simulink model "model_socrates"  (R2019b)
settings: Solver=VariableStepAuto  StartTime=0.0  StopTime=nb_time_unit_in_a_simulation/5  RelTol=1e-3
values from neighbouring files (symbols this model uses):
  nb_air_cons = nb_rooms-2    [load_parameters.m]
  nb_boilers = 2    [load_parameters.m]
  nb_radiators = nb_rooms-2    [load_parameters.m]
  nb_second_in_timeunit = 60*5    (= 300)    [full_test.m]
  nb_step_to_fifteen_min = 3    [full_test.m]
  nb_step_to_one_h = 12    [full_test.m]
  nb_step_to_thirty_min = 6    [full_test.m]
  timeunit_in_a_day = 2*6*24    (= 288)    [full_test.m]
undefined symbols (not defined in the file or in its folder): air_mass_kg_rooms, Area_boiler, area_outdoor_rooms, Area_radiators, area_rooms_ground, area_walls_between_rooms, C_air, C_water, Energy_used_by_air_conditioner_for_1_timeunit_in_Watts_vector, Energy_used_by_air_mixer_for_1_timeunit_in_Watts, Energy_used_by_boiler_for_1_timeunit_in_Watts, initial_relative_humidity, initial_temp_water_in_boilers, initial_temperature_rooms, initial_temperature_water_in_radiator, k_boiler_border, k_radiators, k_wall_outdoor_rooms, k_walls_between_rooms, mass_water_radiator, matrix_AC_rooms_locations, matrix_boiler_radiator_connection, matrix_boiler_rooms_locations, matrix_radiator_rooms_locations, nb_humans, nb_rooms, outdoor_max_temp_A, outdoor_max_temp_B, outdoor_min_temp_A, outdoor_min_temp_B, tau_boiler, thickness_boiler, thickness_outdoor_rooms, thickness_radiator_pipes, thickness_walls_between_rooms, Volume_radiators, Volume_rooms, water_weight_in_boiler, watt_generation_of_employe
libraries: dspmtrx3 x15, dspstat3 x6, simulink x2
(part 1 of 2)
settings Model: Creator=pat  LastModifiedBy=pat

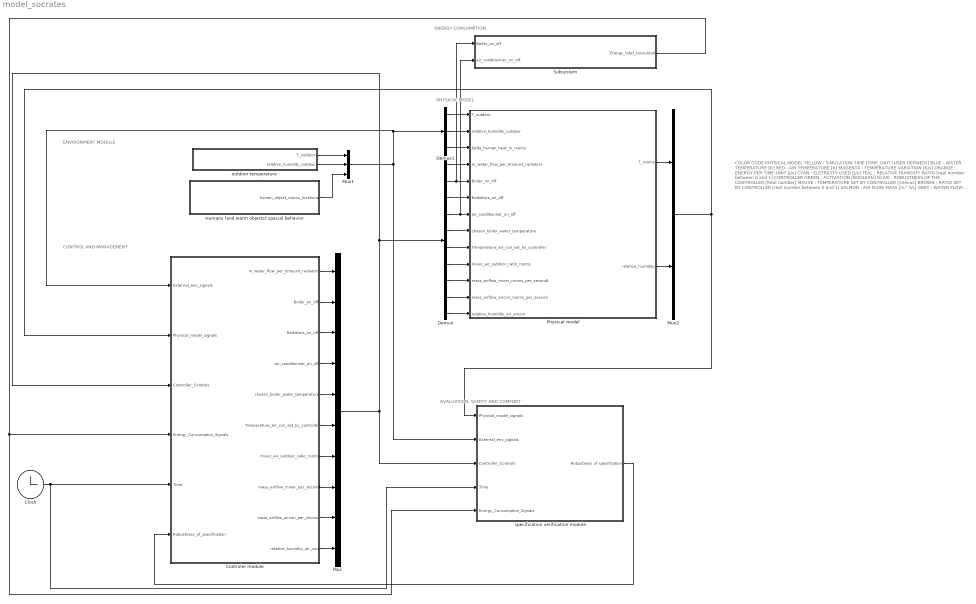
== system model_socrates ==
  note: EVALUATION, SAFETY AND COMFORT
  note: PHYSICAL MODEL
  note: ENVIRONMENT MODULE
  note: COLOR CODE
      |
      | PHYSICAL MODEL
      |
      | YELLOW : SIMULATION TIME [TIME_UNIT (USER DEFINED)]
      | BLUE : WATER TEMPERATURE [K]
      | RED : AIR TEMPERATURE [K]
      | MAGENTA : TEMPERATURE VARIATION [K/s]
      | ORANGE : ENERGY PER TIME-UNIT [J/s]
      | CYAN : ELETRICITY USED [J/s]
      | TEAL : RELATIVE HUMIDITY RATIO [real number between 0 and 1]
      |
      | CONTROLLER
      |
      | GREEN : ACTIVATION [BOOLEAN]
      | OLIVE : ROBUSTNESS OF THE CONTROLLER [Real number]
      | MAUVE : TEMPERATURE SET BY CONTROLLER [Celsius]
      | BROWN : RATIO SET BY CONTROLLER [real number between 0 and 1]
      | SALMON : AIR FLOW MASS [m^3/s]
      | GREY : WATER FLOW MASS [m^3/s]
      |
      | ENVIRONMENT STOCHASTIC BEHAVIORS
      |
      | PURPLE : WARM HUMAN AND OBJECTS LOCATION
      | : POSSESES SOME STOCHASTIC BEHAVIORS
  note: CONTROL AND MANAGEMENT
  note: ENERGY CONSUMPTION
  Clock : Clock
  Controler module : Subsystem
  Demux : Demux  Outputs=[nb_radiators nb_boilers nb_radiators nb_air_cons nb_boilers nb_air_cons nb_rooms nb_rooms nb_air_cons nb_air_cons]
  Demux1 : Demux  Outputs=[1 1 nb_humans]
  "Humans (and warm objects) spacial behavior " : Subsystem
  Mux : Mux  Inputs=10
  Mux1 : Mux  Inputs=3
  Mux2 : Mux  Inputs=2
  Physical model : Subsystem
  Subsystem : Subsystem
  outdoor temperature : Subsystem
  specification verification module : Subsystem
  wires:
  specification verification module/1(Robustness of spesification) -> Controler module/6(Robustness_of_specification)
  Physical model/2(relative_humidity) -> Mux2/2
  Controler module/1(m_water_flow_per_timeunit_radiators) -> Mux/1
  Controler module/2(Boiler_on_off) -> Mux/2
  Controler module/3(Radiators_on_off) -> Mux/3
  Controler module/4(air_conditionner_on_off) -> Mux/4
  Controler module/5(chosen_boiler_water_temperature) -> Mux/5
  Controler module/6(Temperature_air_con_set_by_controller) -> Mux/6
  Controler module/7("mixer_air_outdoor_ratio_rooms ") -> Mux/7
  Controler module/8(mass_airflow_mixer_per_second) -> Mux/8
  Controler module/9(mass_airflow_aircon_per_second) -> Mux/9
  Controler module/10(relative_humidity_air_con) -> Mux/10
  Demux/1 -> Physical model/4(m_water_flow_per_timeunit_radiators)
  Demux/3 -> Physical model/6(Radiators_on_off)
  Demux/10 -> Physical model/13(relative_humidity_air_aircon)
  Demux/9 -> Physical model/12(mass_airflow_aircon_rooms_per_second)
  Demux/8 -> Physical model/11(mass_airflow_mixer_rooms_per_secondt)
  Demux/7 -> Physical model/10("mixer_air_outdoor_ratio_rooms ")
  Demux/6 -> Physical model/9(Temperature_air_con_set_by_controller)
  Demux/5 -> Physical model/8(chosen_boiler_water_temperature)
  Clock/1 -> Controler module/5(Time), specification verification module/4(Time)
  "Humans (and warm objects) spacial behavior "/1("human_object_rooms_locations ") -> Mux1/3
  outdoor temperature/2("relative_humidity_outdoor ") -> Mux1/2
  outdoor temperature/1(T_outdoor) -> Mux1/1
  Demux1/1 -> Physical model/1(T_outdoor)
  Demux1/3 -> Physical model/3("Delta_human_heat_in_rooms ")
  Demux1/2 -> Physical model/2(relative_humidity_outdoor)
  Subsystem/1(Energy_total_consumed) -> specification verification module/5(Energy_Consumption_Signals), Controler module/4(Energy_Consumption_Signals)
  Physical model/1(T_rooms) -> Mux2/1
  Mux2/1 -> Controler module/2(Physical_model_signals), specification verification module/1(Physical_model_signals)
  Mux1/1 -> Controler module/1(External_env_signals), Demux1/1, specification verification module/2(External_env_signals)
  Mux/1 -> Controler module/3("Controller_Controls "), Demux/1, specification verification module/3("Controller_Controls ")
  Demux/2 -> Subsystem/1(Boiler_on_off), Physical model/5(Boiler_on_off)
  Demux/4 -> Subsystem/2(air_conditionner_on_off), Physical model/7(air_conditionner_on_off)

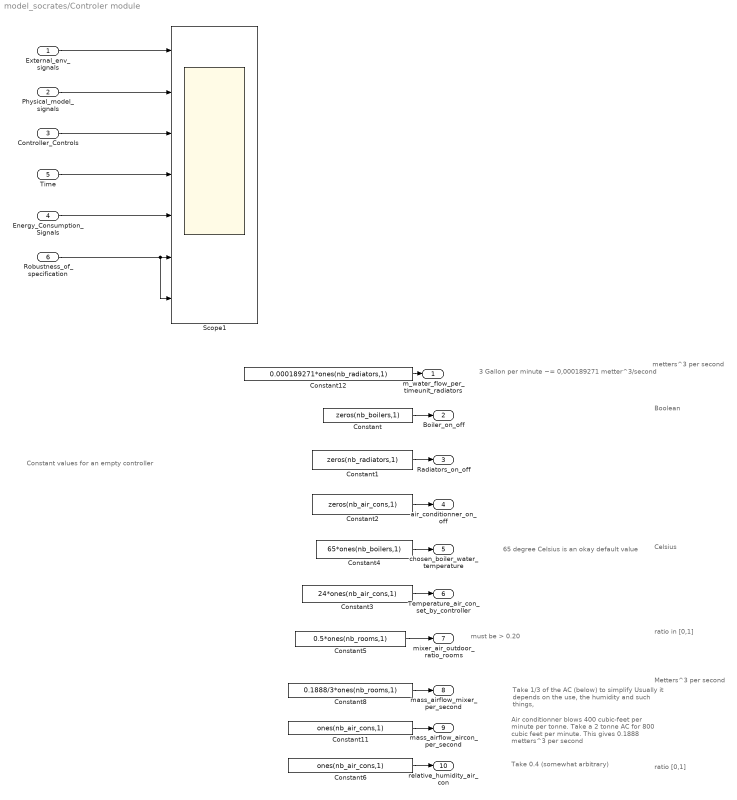
== system model_socrates/Controler module ==
  note: Metters^3 per second
  note: Air conditionner blows 400 cubic-feet per minute per tonne. Take a 2 tonne AC for 800 cubic feet per minute.
      |
      | This gives 0.1888 metters^3 per second
  note: 3 Gallon per minute ~= 0,000189271 metter^3/second
  note: 65 degree Celsius is an okay default value
  note: Constant values
      | for an empty controller
  note: must be > 0.20
  note: Take 1/3 of the AC (below) to simplify
      | Usually it depends on the use, the humidity
      | and such things,
  note: ratio in [0,1]
  note: Celsius
  note: Boolean
  note: metters^3 per second
  note: Take 0.4 (somewhat arbitrary)
  note: ratio [0,1]
  External_env_signals : Inport
  Physical_model_signals : Inport  Port=2
  "Controller_Controls " : Inport  Port=3
  Energy_Consumption_Signals : Inport  Port=4
  Time : Inport  Port=5
  Robustness_of_specification : Inport  Port=6
  Constant : Constant  Value=zeros(nb_boilers,1)
  Constant1 : Constant  Value=zeros(nb_radiators,1)
  Constant11 : Constant  Value=ones(nb_air_cons,1)
  Constant12 : Constant  Value=0.000189271*ones(nb_radiators,1)
  Constant2 : Constant  Value=zeros(nb_air_cons,1)
  Constant3 : Constant  Value=24*ones(nb_air_cons,1)
  Constant4 : Constant  Value=65*ones(nb_boilers,1)
  Constant5 : Constant  Value=0.5*ones(nb_rooms,1)
  Constant6 : Constant  Value=ones(nb_air_cons,1)
  Constant8 : Constant  Value=0.1888/3*ones(nb_rooms,1)
  Scope1 : Scope  NumInputPorts=7
  m_water_flow_per_timeunit_radiators : Outport
  Boiler_on_off : Outport  Port=2
  Radiators_on_off : Outport  Port=3
  air_conditionner_on_off : Outport  Port=4
  chosen_boiler_water_temperature : Outport  Port=5
  Temperature_air_con_set_by_controller : Outport  Port=6
  "mixer_air_outdoor_ratio_rooms " : Outport  Port=7
  mass_airflow_mixer_per_second : Outport  Port=8
  mass_airflow_aircon_per_second : Outport  Port=9
  relative_humidity_air_con : Outport  Port=10
  wires:
  Constant12/1 -> m_water_flow_per_timeunit_radiators/1
  Constant5/1 -> "mixer_air_outdoor_ratio_rooms "/1
  Constant8/1 -> mass_airflow_mixer_per_second/1
  Constant11/1 -> mass_airflow_aircon_per_second/1
  Constant3/1 -> Temperature_air_con_set_by_controller/1
  Constant4/1 -> chosen_boiler_water_temperature/1
  Constant/1 -> Boiler_on_off/1
  Constant1/1 -> Radiators_on_off/1
  Constant2/1 -> air_conditionner_on_off/1
  Constant6/1 -> relative_humidity_air_con/1
  External_env_signals/1 -> Scope1/1
  Physical_model_signals/1 -> Scope1/2
  "Controller_Controls "/1 -> Scope1/3
  Time/1 -> Scope1/4
  Energy_Consumption_Signals/1 -> Scope1/5
  Robustness_of_specification/1 -> Scope1/7, Scope1/6

== system model_socrates/Humans (and warm objects) spacial behavior  ==
  From File : FromFile  FileName=Model_files/matlab_format_input_data/huma_locations.mat  SampleTime=0
  Uniform Random Number : UniformRandomNumber  Commented=on  Minimum=ones(nb_humans,1)  Maximum=nb_rooms*ones(nb_humans,1)  Seed=[1:nb_humans]  SampleTime=60*6
  "human_object_rooms_locations " : Outport
  wires:
  From File/1 -> "human_object_rooms_locations "/1

== system model_socrates/Physical model ==
  note: HUMIDITY EVOLUTION
  note: BOILER AND RADIATORS
  note: AIR FLOW MOVMENTS
      | 								  gives the new temperature after injection of the new air from mixer and ventilation
  note: ROOM TEMPERATURE EVOLUTIONS
  note: WALL HEAT EXCHANGE
  T_outdoor : Inport
  relative_humidity_outdoor : Inport  Port=2
  "Delta_human_heat_in_rooms " : Inport  Port=3
  m_water_flow_per_timeunit_radiators : Inport  Port=4
  Boiler_on_off : Inport  Port=5
  Radiators_on_off : Inport  Port=6
  air_conditionner_on_off : Inport  Port=7
  chosen_boiler_water_temperature : Inport  Port=8
  Temperature_air_con_set_by_controller : Inport  Port=9
  "mixer_air_outdoor_ratio_rooms " : Inport  Port=10
  mass_airflow_mixer_rooms_per_secondt : Inport  Port=11
  mass_airflow_aircon_rooms_per_second : Inport  Port=12
  relative_humidity_air_aircon : Inport  Port=13
  Air conditionning : Subsystem
  "Air mixer temperature (air from outside mixed with current room air) " : Subsystem
  Boiler_contour_heat_exchange : Subsystem
  Human heat exchange : Subsystem
  Radiator heat Exchange : Subsystem
  Subsystem : Subsystem
  Temperature variation in rooms : Subsystem
  Temperature water in boiler : Subsystem
  Wall heat Exchange module : Subsystem
  T_rooms : Outport
  relative_humidity : Outport  Port=2
  wires:
  Boiler_contour_heat_exchange/1(Delta_boiler_room_to_boiler_water) -> Temperature water in boiler/1(Delta_boiler_room_to_boiler)
  Temperature_air_con_set_by_controller/1 -> Air conditionning/2(Temperature_air_con_set_by_controller)
  T_outdoor/1 -> "Air mixer temperature (air from outside mixed with current room air) "/2(T_outdoor), Wall heat Exchange module/2(T_outdoor)
  "mixer_air_outdoor_ratio_rooms "/1 -> "Air mixer temperature (air from outside mixed with current room air) "/3("mixer_air_outdoor_ratio_rooms ")
  Temperature variation in rooms/1(T_rooms) -> T_rooms/1, Wall heat Exchange module/1(T_rooms), Radiator heat Exchange/4(T_rooms), "Air mixer temperature (air from outside mixed with current room air) "/1(T_rooms), Boiler_contour_heat_exchange/2(T_rooms)
  chosen_boiler_water_temperature/1 -> Temperature water in boiler/2(chosen_boiler_water_temperature)
  Boiler_on_off/1 -> Temperature water in boiler/3(Boiler_on_off)
  Temperature water in boiler/1(temperature_water_in_boiler) -> Radiator heat Exchange/1(temperature_water_in_boiler), Boiler_contour_heat_exchange/1(temperature_water_in_boilers)
  "Air mixer temperature (air from outside mixed with current room air) "/1("T_mixer_rooms ") -> Temperature variation in rooms/8("T_mixer_rooms ")
  Air conditionning/1(T_air_cons) -> Temperature variation in rooms/9(T_air_cons)
  Wall heat Exchange module/1("Delta_wall_rooms ") -> Temperature variation in rooms/2(Delta_walls/rooms)
  "Delta_human_heat_in_rooms "/1 -> Human heat exchange/1(In1)
  Boiler_contour_heat_exchange/2(Delta_boiler_water_to_boiler_room) -> Temperature variation in rooms/4(Delta_boiler_rooms)
  Radiator heat Exchange/1(Delta_radiator_rooms) -> Temperature variation in rooms/3(Delta_radiators/rooms)
  air_conditionner_on_off/1 -> Air conditionning/1(air_conditionner_on_off), Subsystem/1("air_conditioner_on_off "), Temperature variation in rooms/5(air_conditionner_on_off)
  Radiators_on_off/1 -> Radiator heat Exchange/3(radiator_on_off)
  mass_airflow_mixer_rooms_per_secondt/1 -> Subsystem/2(mass_airflow_mixer_rooms_per_second), Temperature variation in rooms/6(mass_airflow_mixer_rooms_per_second)
  mass_airflow_aircon_rooms_per_second/1 -> Subsystem/3(mass_airflow_aircon_rooms_per_second), Temperature variation in rooms/7("m_aircon_per_second ")
  m_water_flow_per_timeunit_radiators/1 -> Radiator heat Exchange/2(m_water_flow_per_timeunit_radiators)
  Subsystem/1(relative_humidity) -> relative_humidity/1
  relative_humidity_air_aircon/1 -> Subsystem/5(relative humidity new air aircon)
  relative_humidity_outdoor/1 -> Subsystem/4(relative humidity outdoor)
  Human heat exchange/1("Delta_human_heat_in_rooms ") -> Temperature variation in rooms/1(Delta_humans_objects_heat_in_rooms)

== system model_socrates/Subsystem ==
  Boiler_on_off : Inport
  air_conditionner_on_off : Inport  Port=2
  Energy consumption air conditionners (per private rooms) : Subsystem
  Energy consumption air mixer : Subsystem
  Energy consumption boiler : Subsystem
  Sum : Sum  Inputs=|+++
  Sum of Elements : Sum  Inputs=+
  Energy_total_consumed : Outport
  wires:
  Energy consumption boiler/1(Energy_used_by_boiler) -> Sum/1
  Energy consumption air mixer/1(Energy_used_by_air_mixer) -> Sum/3
  Sum/1 -> Energy_total_consumed/1
  Sum of Elements/1 -> Sum/2
  Energy consumption air conditionners (per private rooms)/1(energy_used_by_air_cons_per_private_room_(vector)) -> Sum of Elements/1
  Boiler_on_off/1 -> Energy consumption boiler/1(Boiler_on_off)
  air_conditionner_on_off/1 -> Energy consumption air conditionners (per private rooms)/1(air_conditionner_on_off)

== system model_socrates/outdoor temperature ==
  note: TEMPERATURE
  note: HUMIDITY
  note: OLD MODULE TO CREATE A SINUSOIDAL AND SIMULATE THE EXTERNAL
      | TEMPERATURE AND HUMIDITY.
  note: Description
      | Sinwave lowering randomly in [min_temp_A, min_temp_B] and maxing in [max_temp_A, max_temp_B]. Made for 24 hours then repeat itself.
      |
      | Equation (past the random number generation)
      |
      | $min_{temp}+(max_{temp}-min_{temp})[0.5+0.5sin(\frac{-\pi}{2}-\frac{\pi}{6}+\frac{2\pi t}{tuid})]$
      |
      | where pod corresponds to the number of time unit for one day (if 1unit = 1h then pod=24, if 1unit=1minute then pod=24*60)
  note: Simulation Inputs:
      |
      | min_temp_A : double
      | min_temp_B : double
      | max_temp_A : double
      | max_temp_B : double
      | timeunit_in_a_day : double
  Add : Sum  Commented=on
  From File : FromFile  FileName=Model_files/matlab_format_input_data/external_temperature.mat  SampleTime=0
  From File1 : FromFile  FileName=Model_files/matlab_format_input_data/external_humidity.mat  SampleTime=0
  "Max temeprature of the sinwave random in [max_temp_A, max_temp_B] " : Constant  Commented=on  Value=outdoor_max_temp_A+randi(outdoor_max_temp_B-outdoor_max_temp_A+1)-1
  "Min and initial temperature of the sinwave random in [min_temp_A, min_temp_B] " : Constant  Commented=on  Value=outdoor_min_temp_A+randi(outdoor_min_temp_B-outdoor_min_temp_A+1)-1
  Product : Product  Commented=on
  Scope : Scope  Commented=on  NumInputPorts=2
  Sinusoidal signal : Sin  Commented=on  Amplitude=1/2  Bias=1/2  Frequency=2*pi/timeunit_in_a_day  Phase=-pi/2-pi/6  SampleTime=0
  Subtract : Sum  Commented=on  Inputs=+-
  constant relative humidity (0.75 for Shanghai in summer is relatively realiste) : Constant  Commented=on  Value=0.75
  T_outdoor : Outport
  "relative_humidity_outdoor " : Outport  Port=2
  wires:
  Product/1 -> Add/2
  "Min and initial temperature of the sinwave random in [min_temp_A, min_temp_B] "/1 -> Subtract/2, Add/1
  Sinusoidal signal/1 -> Product/2
  Subtract/1 -> Product/1
  "Max temeprature of the sinwave random in [max_temp_A, max_temp_B] "/1 -> Subtract/1
  Add/1 -> Scope/1
  constant relative humidity (0.75 for Shanghai in summer is relatively realiste)/1 -> Scope/2
  From File1/1 -> "relative_humidity_outdoor "/1
  From File/1 -> T_outdoor/1

== system model_socrates/specification verification module ==
  Physical_model_signals : Inport
  External_env_signals : Inport  Port=2
  "Controller_Controls " : Inport  Port=3
  Time : Inport  Port=4
  Energy_Consumption_Signals : Inport  Port=5
  Array-Vector Multiply : dspmtrx3/Array-Vector Multiply  mode=Mute  saveAsFlag=0  Dimension=1  V_Source=Input port  V_VectFromMask=[0.5 0.25]  roundingMode=Floor  overflowMode=off  firstCoeffSignedness=Auto  firstCoeffDataTypeStr=Inherit: Same word length as input  firstCoeffMin=[]  firstCoeffMax=[]  firstCoeffLastDataTypeStr=Inherit: Same word length as input  prodOutputSignedness=Auto  accumSignedness=Auto  outputSignedness=Auto  outputDataTypeStr=Inherit: Same as product output  outputMin=[]  outputMax=[]  outputLastDataTypeStr=Inherit: Same as product output
      settings: SourceProductName=DSP System Toolbox  SourceProductBaseCode=DS
  Array-Vector Subtract : dspmtrx3/Array-Vector Subtract  Dimension=2  V_Source=Input port  V_VectFromMask=[0.5 0.25]  prodOutputSignedness=Auto  roundingMode=Floor  overflowMode=off  firstCoeffSignedness=Auto  firstCoeffDataTypeStr=Inherit: Same word length as input  firstCoeffMin=[]  firstCoeffMax=[]  firstCoeffLastDataTypeStr=Inherit: Same word length as input  accumSignedness=Auto  outputSignedness=Auto  outputDataTypeStr=Inherit: Same as accumulator  outputMin=[]  outputMax=[]  outputLastDataTypeStr=Inherit: Same as accumulator
      settings: SourceProductName=DSP System Toolbox  SourceProductBaseCode=DS
  Compare To Constant : simulink/Logic and Bit Operations/Compare To Constant  relop===  const=0  OutDataTypeStr=boolean
  Constant : Constant  Value=area_rooms_ground
  Constant2 : Constant  Value=ones(nb_rooms,nb_humans)
  Demux : Demux  Outputs=[nb_rooms nb_rooms]
  Demux1 : Demux  Outputs=[(2*(nb_boilers+nb_radiators+nb_air_cons))+nb_rooms nb_rooms nb_air_cons*2]
  Demux2 : Demux  Outputs=[2 nb_humans]
  Min : MinMax
  Mux : Mux  Inputs=6
  Subsystem : Subsystem
  Sum of Elements : Sum  Inputs=+  CollapseMode=Specified dimension  CollapseDim=2  OutDataTypeStr=double
  Terminator{,1..4} (5 alike) : Terminator
  rooms : Constant  Value=[1:nb_rooms]
  Robustness of spesification : Outport
  wires:
  Subsystem/1(Out5) -> Mux/1
  Subsystem/2(Out1) -> Mux/2
  Subsystem/3(Out2) -> Mux/3
  Subsystem/4(Out3) -> Mux/4
  Subsystem/5(Out4) -> Mux/5
  Physical_model_signals/1 -> Demux/1
  Demux/1 -> Subsystem/4(T_rooms)
  Demux/2 -> Subsystem/5(RH_rooms)
  External_env_signals/1 -> Demux2/1
  Constant/1 -> Subsystem/2(Area_rooms)
  Array-Vector Subtract/1 -> Compare To Constant/1
  Array-Vector Multiply/1 -> Array-Vector Subtract/1
  Compare To Constant/1 -> Sum of Elements/1
  rooms/1 -> Array-Vector Multiply/2
  Constant2/1 -> Array-Vector Multiply/1
  Demux2/2 -> Array-Vector Subtract/2
  Sum of Elements/1 -> Subsystem/3(nb_person_in_rooms)  "nb human in room"
  Demux1/2 -> Subsystem/1(ventilation_airflow_outdoor_air_mcube_rooms)
  "Controller_Controls "/1 -> Demux1/1
  Subsystem/6(Out6) -> Mux/6
  Demux1/1 -> Terminator/1
  Demux1/3 -> Terminator1/1
  Demux2/1 -> Terminator2/1
  Time/1 -> Terminator4/1
  Energy_Consumption_Signals/1 -> Terminator3/1
  Min/1 -> Robustness of spesification/1
  Mux/1 -> Min/1

== system model_socrates/Physical model/Air conditionning ==
  note: For this experiment, we assume that the air blown by the air conditionner is immediatly
      | set to the temperature chosen in the controller.
      |
      | People that wants a "ramp up" (or ramp down) the air blown upon activation can add some blocks here.
  air_conditionner_on_off : Inport
  Temperature_air_con_set_by_controller : Inport  Port=2
  Scope : Scope
  T_air_cons : Outport
  wires:
  Temperature_air_con_set_by_controller/1 -> T_air_cons/1
  air_conditionner_on_off/1 -> Scope/1

== system model_socrates/Physical model/Air mixer temperature (air from outside mixed with current room air)  ==
  note: Simulation Parameters :
      | mix_ratio (% new from outside air) : double in [0,1]
  note: Evolution of the air temperature T_d in the air mixer and ventilation system.
      | The temperature follows the equation below
      |
      | $T(t)=mix.ratio*T_{outdoor}(t)+(1-mix.ratio)*T(t)$
  T_rooms : Inport
  T_outdoor : Inport  Port=2
  "mixer_air_outdoor_ratio_rooms " : Inport  Port=3
  Constant : Constant
  Product : Product
  Product3 : Product
  Subtract : Sum  Inputs=+-
  Sum : Sum  Inputs=|++
  "T_mixer_rooms " : Outport
  wires:
  T_rooms/1 -> Product/1
  Product/1 -> Sum/1
  Sum/1 -> "T_mixer_rooms "/1
  Product3/1 -> Sum/2
  Constant/1 -> Subtract/1
  Subtract/1 -> Product3/1
  "mixer_air_outdoor_ratio_rooms "/1 -> Product/2, Subtract/2
  T_outdoor/1 -> Product3/2

== system model_socrates/Physical model/Boiler_contour_heat_exchange ==
  note: heat transfer from the boiler water to the boiler room
  temperature_water_in_boilers : Inport
  T_rooms : Inport  Port=2
  Array-Vector Multiply1 : dspmtrx3/Array-Vector Multiply  mode=Mute  saveAsFlag=0  Dimension=1  V_Source=Input port  V_VectFromMask=[0.5 0.25]  roundingMode=Floor  overflowMode=off  firstCoeffSignedness=Auto  firstCoeffDataTypeStr=Inherit: Same word length as input  firstCoeffMin=[]  firstCoeffMax=[]  firstCoeffLastDataTypeStr=Inherit: Same word length as input  prodOutputSignedness=Auto  accumSignedness=Auto  outputSignedness=Auto  outputDataTypeStr=Inherit: Same as product output  outputMin=[]  outputMax=[]  outputLastDataTypeStr=Inherit: Same as product output
      settings: SourceProductName=DSP System Toolbox  SourceProductBaseCode=DS
  Array-Vector Multiply2 : dspmtrx3/Array-Vector Multiply  mode=Mute  saveAsFlag=0  Dimension=2  V_Source=Input port  V_VectFromMask=[0.5 0.25]  roundingMode=Floor  overflowMode=off  firstCoeffSignedness=Auto  firstCoeffDataTypeStr=Inherit: Same word length as input  firstCoeffMin=[]  firstCoeffMax=[]  firstCoeffLastDataTypeStr=Inherit: Same word length as input  prodOutputSignedness=Auto  accumSignedness=Auto  outputSignedness=Auto  outputDataTypeStr=Inherit: Same as product output  outputMin=[]  outputMax=[]  outputLastDataTypeStr=Inherit: Same as product output
      settings: SourceProductName=DSP System Toolbox  SourceProductBaseCode=DS
  Constant1 : Constant  Value=matrix_boiler_rooms_locations
  Constant2 : Constant  Value=matrix_boiler_rooms_locations
  Gain : Gain  Gain=-1
  Gain1 : Gain  Gain=ones(nb_boilers,1)./thickness_boiler
  Gain2 : Gain  Gain=1/C_water
  Gain3 : Gain  Gain=1/C_air
  Gain4 : Gain  Gain=k_boiler_border
  Gain5 : Gain  Gain=Area_boiler
  Gain6 : Gain  Gain=ones(1,nb_rooms)./air_mass_kg_rooms
  Gain7 : Gain  Gain=ones(nb_boilers,1)./water_weight_in_boiler
  Sum of Elements : Sum  Inputs=+  CollapseMode=Specified dimension
  Sum of Elements1 : Sum  Inputs=+  CollapseMode=Specified dimension  CollapseDim=2
  Sum1 : Sum  Inputs=|+-
  Delta_boiler_room_to_boiler_water : Outport
  Delta_boiler_water_to_boiler_room : Outport  Port=2
  wires:
  Gain4/1 -> Gain1/1
  Sum1/1 -> Gain4/1
  T_rooms/1 -> Array-Vector Multiply2/2
  Gain5/1 -> Gain3/1, Gain/1
  Gain/1 -> Gain2/1
  Gain2/1 -> Gain7/1
  Gain1/1 -> Gain5/1
  Constant2/1 -> Array-Vector Multiply2/1
  Array-Vector Multiply2/1 -> Sum of Elements1/1
  temperature_water_in_boilers/1 -> Sum1/1
  Sum of Elements1/1 -> Sum1/2
  Gain7/1 -> Delta_boiler_room_to_boiler_water/1
  Array-Vector Multiply1/1 -> Sum of Elements/1
  Constant1/1 -> Array-Vector Multiply1/1
  Sum of Elements/1 -> Gain6/1
  Gain3/1 -> Array-Vector Multiply1/2
  Gain6/1 -> Delta_boiler_water_to_boiler_room/1

== system model_socrates/Physical model/Human heat exchange ==
  note: Numbers vary from 50 to 100 J/s
  note: if timeunit is not a second, the change is handled at then end of the pipe.
      |
      | no worry
  In1 : Inport
  Array-Vector Multiply : dspmtrx3/Array-Vector Multiply  mode=Mute  saveAsFlag=0  Dimension=1  V_Source=Input port  V_VectFromMask=[0.5 0.25]  roundingMode=Floor  overflowMode=off  firstCoeffSignedness=Auto  firstCoeffDataTypeStr=Inherit: Same word length as input  firstCoeffMin=[]  firstCoeffMax=[]  firstCoeffLastDataTypeStr=Inherit: Same word length as input  prodOutputSignedness=Auto  accumSignedness=Auto  outputSignedness=Auto  outputDataTypeStr=Inherit: Same as product output  outputMin=[]  outputMax=[]  outputLastDataTypeStr=Inherit: Same as product output
      settings: SourceProductName=DSP System Toolbox  SourceProductBaseCode=DS
  Array-Vector Subtract : dspmtrx3/Array-Vector Subtract  Dimension=2  V_Source=Input port  V_VectFromMask=[0.5 0.25]  prodOutputSignedness=Auto  roundingMode=Floor  overflowMode=off  firstCoeffSignedness=Auto  firstCoeffDataTypeStr=Inherit: Same word length as input  firstCoeffMin=[]  firstCoeffMax=[]  firstCoeffLastDataTypeStr=Inherit: Same word length as input  accumSignedness=Auto  outputSignedness=Auto  outputDataTypeStr=Inherit: Same as accumulator  outputMin=[]  outputMax=[]  outputLastDataTypeStr=Inherit: Same as accumulator
      settings: SourceProductName=DSP System Toolbox  SourceProductBaseCode=DS
  Compare To Constant : simulink/Logic and Bit Operations/Compare To Constant  relop===  const=0  OutDataTypeStr=boolean
  Constant2 : Constant  Value=ones(nb_rooms,nb_humans)
  Gain3 : Gain  Gain=1/C_air
  Gain6 : Gain  Gain=ones(nb_rooms,1)./air_mass_kg_rooms
  Sum of Elements : Sum  Inputs=+  CollapseMode=Specified dimension  CollapseDim=2
  Watts production per sec (estimation) : Gain  Gain=watt_generation_of_employe
  rooms : Constant  Value=[1:nb_rooms]
  "Delta_human_heat_in_rooms " : Outport
  wires:
  Compare To Constant/1 -> Sum of Elements/1
  rooms/1 -> Array-Vector Multiply/2
  Sum of Elements/1 -> Watts production per sec (estimation)/1  "nb human in room"
  Array-Vector Multiply/1 -> Array-Vector Subtract/1
  Watts production per sec (estimation)/1 -> Gain6/1
  Gain6/1 -> Gain3/1
  Gain3/1 -> "Delta_human_heat_in_rooms "/1
  Array-Vector Subtract/1 -> Compare To Constant/1
  Constant2/1 -> Array-Vector Multiply/1
  In1/1 -> Array-Vector Subtract/2

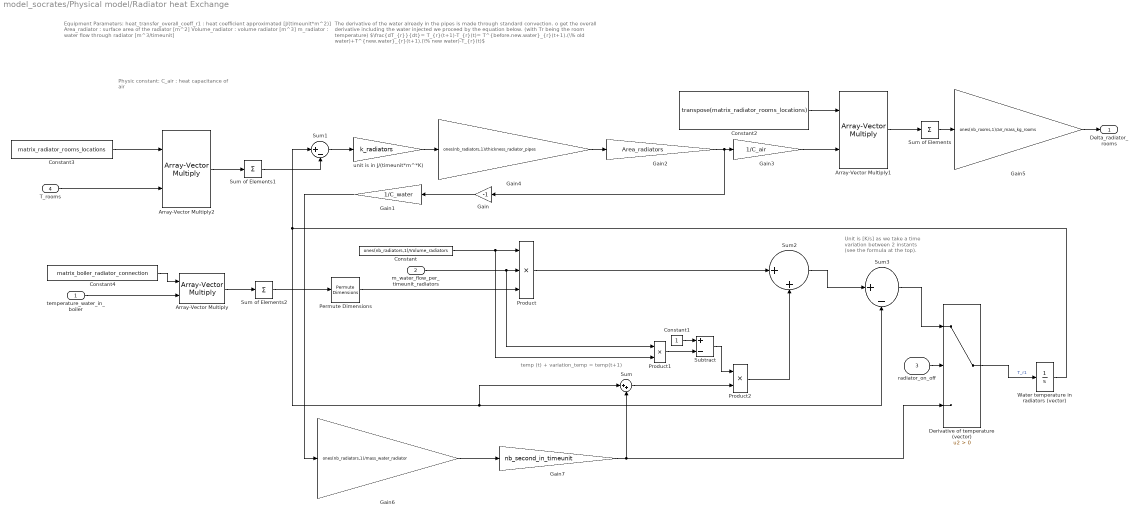
== system model_socrates/Physical model/Radiator heat Exchange ==
  note: Unit is [K/s] as we take a time
      | variation between 2 instants
      | (see the formula at the top).
  note: Physic constant:
      | C_air : heat capacitance of air
  note: Equipment Parameters:
      | heat_transfer_overall_coeff_r1 : heat coefficient approximated [J/(timeunit*m^2)]
      | Area_radiator : surface area of the radiator [m^2]
      | Volume_radiator : volume radiator [m^3]
      | m_radiator : water flow through radiator [m^3/timeunit]
  note: The derivative of the water already in the pipes is made through standard convection. o get the overall derivative including the water injected we proceed by the equation below. (with
      | Tr being the room temperature)
      |
      | $\frac{dT_{r}}{dt}= T_{r}(t+1)-T_{r}(t)= T^{before.new.water}_{r}(t+1).(\% old water)+T^{new.water}_{r}(t+1).(\% new water)-T_{r}(t)$
  note: temp (t) + variation_temp = temp(t+1)
  temperature_water_in_boiler : Inport
  m_water_flow_per_timeunit_radiators : Inport  Port=2
  radiator_on_off : Inport  Port=3
  T_rooms : Inport  Port=4
  Array-Vector Multiply : dspmtrx3/Array-Vector Multiply  mode=Mute  saveAsFlag=0  Dimension=1  V_Source=Input port  V_VectFromMask=[0.5 0.25]  roundingMode=Floor  overflowMode=off  firstCoeffSignedness=Auto  firstCoeffDataTypeStr=Inherit: Same word length as input  firstCoeffMin=[]  firstCoeffMax=[]  firstCoeffLastDataTypeStr=Inherit: Same word length as input  prodOutputSignedness=Auto  accumSignedness=Auto  outputSignedness=Auto  outputDataTypeStr=Inherit: Same as product output  outputMin=[]  outputMax=[]  outputLastDataTypeStr=Inherit: Same as product output
      settings: SourceProductName=DSP System Toolbox  SourceProductBaseCode=DS
  Array-Vector Multiply1 : dspmtrx3/Array-Vector Multiply  mode=Mute  saveAsFlag=0  Dimension=2  V_Source=Input port  V_VectFromMask=[0.5 0.25]  roundingMode=Floor  overflowMode=off  firstCoeffSignedness=Auto  firstCoeffDataTypeStr=Inherit: Same word length as input  firstCoeffMin=[]  firstCoeffMax=[]  firstCoeffLastDataTypeStr=Inherit: Same word length as input  prodOutputSignedness=Auto  accumSignedness=Auto  outputSignedness=Auto  outputDataTypeStr=Inherit: Same as product output  outputMin=[]  outputMax=[]  outputLastDataTypeStr=Inherit: Same as product output
      settings: SourceProductName=DSP System Toolbox  SourceProductBaseCode=DS
  Array-Vector Multiply2 : dspmtrx3/Array-Vector Multiply  mode=Mute  saveAsFlag=0  Dimension=2  V_Source=Input port  V_VectFromMask=[0.5 0.25]  roundingMode=Floor  overflowMode=off  firstCoeffSignedness=Auto  firstCoeffDataTypeStr=Inherit: Same word length as input  firstCoeffMin=[]  firstCoeffMax=[]  firstCoeffLastDataTypeStr=Inherit: Same word length as input  prodOutputSignedness=Auto  accumSignedness=Auto  outputSignedness=Auto  outputDataTypeStr=Inherit: Same as product output  outputMin=[]  outputMax=[]  outputLastDataTypeStr=Inherit: Same as product output
      settings: SourceProductName=DSP System Toolbox  SourceProductBaseCode=DS
  Constant : Constant  Value=ones(nb_radiators,1)/Volume_radiators
  Constant1 : Constant
  Constant2 : Constant  Value=transpose(matrix_radiator_rooms_locations)
  Constant3 : Constant  Value=matrix_radiator_rooms_locations
  Constant4 : Constant  Value=matrix_boiler_radiator_connection
  Derivative of temperature (vector) : Switch  Criteria=u2 > Threshold
  Gain : Gain  Gain=-1
  Gain1 : Gain  Gain=1/C_water
  Gain2 : Gain  Gain=Area_radiators
  Gain3 : Gain  Gain=1/C_air
  Gain4 : Gain  Gain=ones(nb_radiators,1)/thickness_radiator_pipes
  Gain5 : Gain  Gain=ones(nb_rooms,1)/air_mass_kg_rooms
  Gain6 : Gain  Gain=ones(nb_radiators,1)/mass_water_radiator
  Gain7 : Gain  Gain=nb_second_in_timeunit
  Permute Dimensions : PermuteDimensions
  Product : Product  Inputs=3
  Product1 : Product
  Product2 : Product
  Subtract : Sum  Inputs=+-
  Sum : Sum  Inputs=|++
  Sum of Elements : Sum  Inputs=+  CollapseMode=Specified dimension  CollapseDim=2
  Sum of Elements1 : Sum  Inputs=+  CollapseMode=Specified dimension  CollapseDim=2
  Sum of Elements2 : Sum  Inputs=+  CollapseMode=Specified dimension
  Sum1 : Sum  Inputs=|+-
  Sum2 : Sum  Inputs=|++
  Sum3 : Sum  Inputs=|+-
  Water temperature in radiators (vector) : Integrator  InitialCondition=initial_temperature_water_in_radiator
  unit is in J/(timeunit*m^*K) : Gain  Gain=k_radiators
  Delta_radiator_rooms : Outport
  wires:
  Gain2/1 -> Gain/1, Gain3/1
  Sum1/1 -> unit is in J/(timeunit*m^*K)/1
  Gain1/1 -> Gain6/1
  T_rooms/1 -> Array-Vector Multiply2/2
  radiator_on_off/1 -> Derivative of temperature (vector)/2
  temperature_water_in_boiler/1 -> Array-Vector Multiply/2
  unit is in J/(timeunit*m^*K)/1 -> Gain4/1
  Product/1 -> Sum2/1
  Derivative of temperature (vector)/1 -> Water temperature in radiators (vector)/1  "T_r1"
  Gain/1 -> Gain1/1
  Water temperature in radiators (vector)/1 -> Sum1/1, Sum/1, Sum3/2
  Sum2/1 -> Sum3/1
  Sum3/1 -> Derivative of temperature (vector)/1
  Sum/1 -> Product2/2
  Gain3/1 -> Array-Vector Multiply1/2
  m_water_flow_per_timeunit_radiators/1 -> Product1/1, Product/2
  Constant/1 -> Product1/2, Product/1
  Constant1/1 -> Subtract/1
  Product1/1 -> Subtract/2
  Product2/1 -> Sum2/2
  Subtract/1 -> Product2/1
  Gain4/1 -> Gain2/1
  Gain5/1 -> Delta_radiator_rooms/1
  Gain6/1 -> Gain7/1
  Array-Vector Multiply1/1 -> Sum of Elements/1
  Constant2/1 -> Array-Vector Multiply1/1
  Sum of Elements/1 -> Gain5/1
  Constant3/1 -> Array-Vector Multiply2/1
  Array-Vector Multiply2/1 -> Sum of Elements1/1
  Sum of Elements1/1 -> Sum1/2
  Constant4/1 -> Array-Vector Multiply/1
  Array-Vector Multiply/1 -> Sum of Elements2/1
  Sum of Elements2/1 -> Permute Dimensions/1
  Gain7/1 -> Sum/2, Derivative of temperature (vector)/3
  Permute Dimensions/1 -> Product/3

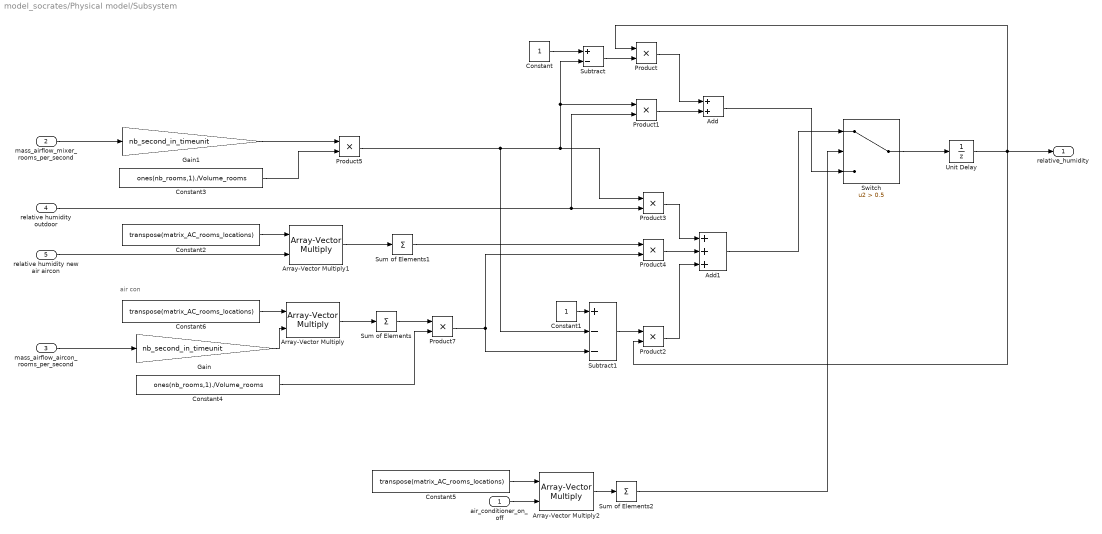
== system model_socrates/Physical model/Subsystem ==
  note: air con
  "air_conditioner_on_off " : Inport
  mass_airflow_mixer_rooms_per_second : Inport  Port=2
  mass_airflow_aircon_rooms_per_second : Inport  Port=3
  relative humidity outdoor : Inport  Port=4
  relative humidity new air aircon : Inport  Port=5
  Add : Sum
  Add1 : Sum  Inputs=+++
  Array-Vector Multiply : dspmtrx3/Array-Vector Multiply  mode=Mute  saveAsFlag=0  Dimension=2  V_Source=Input port  V_VectFromMask=[0.5 0.25]  roundingMode=Floor  overflowMode=off  firstCoeffSignedness=Auto  firstCoeffDataTypeStr=Inherit: Same word length as input  firstCoeffMin=[]  firstCoeffMax=[]  firstCoeffLastDataTypeStr=Inherit: Same word length as input  prodOutputSignedness=Auto  accumSignedness=Auto  outputSignedness=Auto  outputDataTypeStr=Inherit: Same as product output  outputMin=[]  outputMax=[]  outputLastDataTypeStr=Inherit: Same as product output
      settings: SourceProductName=DSP System Toolbox  SourceProductBaseCode=DS
  Array-Vector Multiply1 : dspmtrx3/Array-Vector Multiply  mode=Mute  saveAsFlag=0  Dimension=2  V_Source=Input port  V_VectFromMask=[0.5 0.25]  roundingMode=Floor  overflowMode=off  firstCoeffSignedness=Auto  firstCoeffDataTypeStr=Inherit: Same word length as input  firstCoeffMin=[]  firstCoeffMax=[]  firstCoeffLastDataTypeStr=Inherit: Same word length as input  prodOutputSignedness=Auto  accumSignedness=Auto  outputSignedness=Auto  outputDataTypeStr=Inherit: Same as product output  outputMin=[]  outputMax=[]  outputLastDataTypeStr=Inherit: Same as product output
      settings: SourceProductName=DSP System Toolbox  SourceProductBaseCode=DS
  Array-Vector Multiply2 : dspmtrx3/Array-Vector Multiply  mode=Mute  saveAsFlag=0  Dimension=2  V_Source=Input port  V_VectFromMask=[0.5 0.25]  roundingMode=Floor  overflowMode=off  firstCoeffSignedness=Auto  firstCoeffDataTypeStr=Inherit: Same word length as input  firstCoeffMin=[]  firstCoeffMax=[]  firstCoeffLastDataTypeStr=Inherit: Same word length as input  prodOutputSignedness=Auto  accumSignedness=Auto  outputSignedness=Auto  outputDataTypeStr=Inherit: Same as product output  outputMin=[]  outputMax=[]  outputLastDataTypeStr=Inherit: Same as product output
      settings: SourceProductName=DSP System Toolbox  SourceProductBaseCode=DS
  Constant : Constant
  Constant1 : Constant
  Constant2 : Constant  Value=transpose(matrix_AC_rooms_locations)
  Constant3 : Constant  Value=ones(nb_rooms,1)./Volume_rooms
  Constant4 : Constant  Value=ones(nb_rooms,1)./Volume_rooms
  Constant5 : Constant  Value=transpose(matrix_AC_rooms_locations)
  Constant6 : Constant  Value=transpose(matrix_AC_rooms_locations)
  Gain : Gain  Gain=nb_second_in_timeunit
  Gain1 : Gain  Gain=nb_second_in_timeunit
  Product{,1..5,7} (7 alike) : Product
  Subtract : Sum  Inputs=+-
  Subtract1 : Sum  Inputs=+--
  Sum of Elements : Sum  Inputs=+  CollapseMode=Specified dimension  CollapseDim=2
  Sum of Elements1 : Sum  Inputs=+  CollapseMode=Specified dimension  CollapseDim=2
  Sum of Elements2 : Sum  Inputs=+  CollapseMode=Specified dimension  CollapseDim=2
  Switch : Switch  Criteria=u2 > Threshold  Threshold=0.5
  Unit Delay : UnitDelay  InitialCondition=initial_relative_humidity  SampleTime=-1  HasFrameUpgradeWarning=on
  relative_humidity : Outport
  wires:
  Switch/1 -> Unit Delay/1
  Add/1 -> Switch/3
  Constant/1 -> Subtract/1
  Subtract/1 -> Product/2
  Product/1 -> Add/1
  Product1/1 -> Add/2
  relative humidity outdoor/1 -> Product1/2, Product3/2
  Unit Delay/1 -> Product2/2, Product/1, relative_humidity/1
  Product2/1 -> Add1/3
  Subtract1/1 -> Product2/1
  Constant1/1 -> Subtract1/1
  Add1/1 -> Switch/1
  Product5/1 -> Subtract/2, Product1/1, Product3/1, Subtract1/2
  Product3/1 -> Add1/1
  Product4/1 -> Add1/2
  Product7/1 -> Product4/2, Subtract1/3
  relative humidity new air aircon/1 -> Array-Vector Multiply1/2
  mass_airflow_mixer_rooms_per_second/1 -> Gain1/1
  Gain1/1 -> Product5/1
  Constant3/1 -> Product5/2
  Array-Vector Multiply/1 -> Sum of Elements/1
  Constant6/1 -> Array-Vector Multiply/1
  mass_airflow_aircon_rooms_per_second/1 -> Gain/1
  Gain/1 -> Array-Vector Multiply/2
  Constant4/1 -> Product7/2
  Sum of Elements/1 -> Product7/1
  Constant2/1 -> Array-Vector Multiply1/1
  Array-Vector Multiply1/1 -> Sum of Elements1/1
  Sum of Elements1/1 -> Product4/1
  Sum of Elements2/1 -> Switch/2
  "air_conditioner_on_off "/1 -> Array-Vector Multiply2/2
  Constant5/1 -> Array-Vector Multiply2/1
  Array-Vector Multiply2/1 -> Sum of Elements2/1

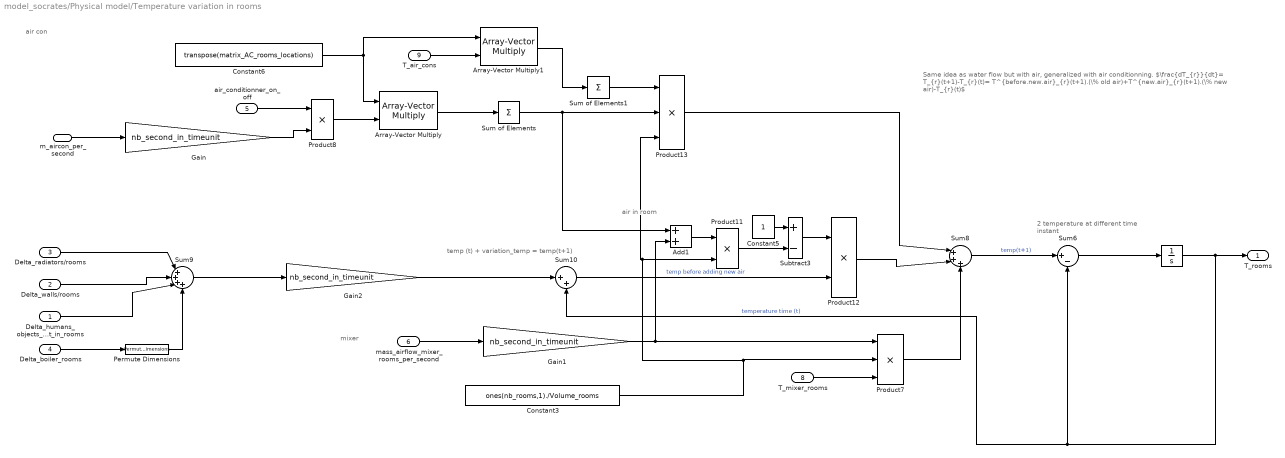
== system model_socrates/Physical model/Temperature variation in rooms ==
  note: air in room
  note: mixer
  note: 2 temperature at
      |  different time instant
  note: temp (t) + variation_temp = temp(t+1)
  note: air con
  note: Same idea as water flow but with air, generalized with air conditionning.
      |
      | $\frac{dT_{r}}{dt}= T_{r}(t+1)-T_{r}(t)= T^{before.new.air}_{r}(t+1).(\% old air)+T^{new.air}_{r}(t+1).(\% new air)-T_{r}(t)$
  Delta_humans_objects_heat_in_rooms : Inport
  Delta_walls/rooms : Inport  Port=2
  Delta_radiators/rooms : Inport  Port=3
  Delta_boiler_rooms : Inport  Port=4
  air_conditionner_on_off : Inport  Port=5
  mass_airflow_mixer_rooms_per_second : Inport  Port=6
  "m_aircon_per_second " : Inport  Port=7
  "T_mixer_rooms " : Inport  Port=8
  T_air_cons : Inport  Port=9
  "     " : Integrator  InitialCondition=initial_temperature_rooms
  Add1 : Sum
  Array-Vector Multiply : dspmtrx3/Array-Vector Multiply  mode=Mute  saveAsFlag=0  Dimension=2  V_Source=Input port  V_VectFromMask=[0.5 0.25]  roundingMode=Floor  overflowMode=off  firstCoeffSignedness=Auto  firstCoeffDataTypeStr=Inherit: Same word length as input  firstCoeffMin=[]  firstCoeffMax=[]  firstCoeffLastDataTypeStr=Inherit: Same word length as input  prodOutputSignedness=Auto  accumSignedness=Auto  outputSignedness=Auto  outputDataTypeStr=Inherit: Same as product output  outputMin=[]  outputMax=[]  outputLastDataTypeStr=Inherit: Same as product output
      settings: SourceProductName=DSP System Toolbox  SourceProductBaseCode=DS
  Array-Vector Multiply1 : dspmtrx3/Array-Vector Multiply  mode=Mute  saveAsFlag=0  Dimension=2  V_Source=Input port  V_VectFromMask=[0.5 0.25]  roundingMode=Floor  overflowMode=off  firstCoeffSignedness=Auto  firstCoeffDataTypeStr=Inherit: Same word length as input  firstCoeffMin=[]  firstCoeffMax=[]  firstCoeffLastDataTypeStr=Inherit: Same word length as input  prodOutputSignedness=Auto  accumSignedness=Auto  outputSignedness=Auto  outputDataTypeStr=Inherit: Same as product output  outputMin=[]  outputMax=[]  outputLastDataTypeStr=Inherit: Same as product output
      settings: SourceProductName=DSP System Toolbox  SourceProductBaseCode=DS
  Constant3 : Constant  Value=ones(nb_rooms,1)./Volume_rooms
  Constant5 : Constant
  Constant6 : Constant  Value=transpose(matrix_AC_rooms_locations)
  Gain : Gain  Gain=nb_second_in_timeunit
  Gain1 : Gain  Gain=nb_second_in_timeunit
  Gain2 : Gain  Gain=nb_second_in_timeunit
  Permute Dimensions : PermuteDimensions
  Product11 : Product
  Product12 : Product
  Product13 : Product  Inputs=3
  Product7 : Product  Inputs=3
  Product8 : Product
  Subtract3 : Sum  Inputs=+-
  Sum of Elements : Sum  Inputs=+  CollapseMode=Specified dimension  CollapseDim=2
  Sum of Elements1 : Sum  Inputs=+  CollapseMode=Specified dimension  CollapseDim=2
  Sum10 : Sum  Inputs=|++
  Sum6 : Sum  Inputs=|+-
  Sum8 : Sum  Inputs=|+++
  Sum9 : Sum  Inputs=|++++
  T_rooms : Outport
  wires:
  Product11/1 -> Subtract3/2
  Product12/1 -> Sum8/2
  Delta_walls/rooms/1 -> Sum9/2
  Subtract3/1 -> Product12/1
  "T_mixer_rooms "/1 -> Product7/3
  Add1/1 -> Product11/1
  mass_airflow_mixer_rooms_per_second/1 -> Gain1/1
  Delta_radiators/rooms/1 -> Sum9/1
  "m_aircon_per_second "/1 -> Gain/1
  "     "/1 -> T_rooms/1, Sum6/2, Sum10/2  "temperature time (t)"
  Sum6/1 -> "     "/1
  Sum10/1 -> Product12/2  "temp before adding new air"
  Constant3/1 -> Product7/2, Product11/2, Product13/3
  Sum9/1 -> Gain2/1
  Delta_humans_objects_heat_in_rooms/1 -> Sum9/3
  Delta_boiler_rooms/1 -> Permute Dimensions/1
  Product7/1 -> Sum8/3
  Sum8/1 -> Sum6/1  "temp(t+1)"
  Constant5/1 -> Subtract3/1
  Constant6/1 -> Array-Vector Multiply1/1, Array-Vector Multiply/1
  Array-Vector Multiply/1 -> Sum of Elements/1
  Sum of Elements/1 -> Product13/2, Add1/1
  T_air_cons/1 -> Array-Vector Multiply1/2
  Product13/1 -> Sum8/1
  Product8/1 -> Array-Vector Multiply/2
  air_conditionner_on_off/1 -> Product8/1
  Sum of Elements1/1 -> Product13/1
  Array-Vector Multiply1/1 -> Sum of Elements1/1
  Gain/1 -> Product8/2
  Gain1/1 -> Product7/1, Add1/2
  Gain2/1 -> Sum10/1
  Permute Dimensions/1 -> Sum9/4

== system model_socrates/Physical model/Temperature water in boiler ==
  note: Evolution of the temperature inside the boiler
  note: Simulation input:
      |
      | - cbwt (input 3) is the temperature while running inside the boiler, past loading time (we can choose it via the controller among a range determined by the equipment).
      | IF cbwt-T_water > 0, boiler's water temperature rises
      | IF cbwt-T_water < 0, boiler's water temperature drops
      |
      | Equipment input:
      |
      | - tau_boiler : thermal time constante : double (in timeunit i.e. second/hours/days....)
      |
      | Physic constant:
      | C_water : heat capacitance of water
  note: The boiler temperature follows the equation below when activated
      |
      | $dT_{sw,b}(t)=\frac{kb-T_{sw,b}(t)}{\tau_{sw}}dt$
      |
      | The boiler be either on or of (B_on) based on the controller.
      | - If it is open, then the temperature of the water supply is leaning toward kb_on
      | - If it is closed, then the heat exchange is in conduction.
  Delta_boiler_room_to_boiler : Inport
  chosen_boiler_water_temperature : Inport  Port=2
  Boiler_on_off : Inport  Port=3
  Add : Sum
  Constant : Constant  Value=ones(nb_boilers,1)
  Gain : Gain  Gain=nb_second_in_timeunit
  Gain1 : Gain  Gain=ones(nb_boilers,1)/tau_boiler
  Gain2 : Gain  Gain=nb_second_in_timeunit
  Integrator : Integrator  InitialCondition=initial_temp_water_in_boilers
  Product : Product
  Product1 : Product
  Subtract : Sum  Inputs=+-
  Subtract1 : Sum  Inputs=+-
  temperature_water_in_boiler : Outport  VectorParamsAs1DForOutWhenUnconnected=off
  wires:
  Boiler_on_off/1 -> Product1/2, Subtract1/2
  Add/1 -> Integrator/1
  Integrator/1 -> temperature_water_in_boiler/1, Subtract/2
  Gain1/1 -> Gain/1
  chosen_boiler_water_temperature/1 -> Subtract/1
  Subtract/1 -> Gain1/1
  Delta_boiler_room_to_boiler/1 -> Gain2/1
  Constant/1 -> Subtract1/1
  Subtract1/1 -> Product/1
  Product/1 -> Add/2
  Product1/1 -> Add/1
  Gain/1 -> Product1/1
  Gain2/1 -> Product/2

== system model_socrates/Physical model/Wall heat Exchange module ==
  T_rooms : Inport
  T_outdoor : Inport  Port=2
  Gain1 : Gain  Gain=1/C_air
  Gain7 : Gain  Gain=ones(nb_rooms,1)./air_mass_kg_rooms
  Sum2 : Sum  Inputs=|++
  "Value heat exchange outdoor -> rooms" : Subsystem
  Value heat exchange within building : Subsystem
  "Delta_wall_rooms " : Outport
  wires:
  Gain1/1 -> Gain7/1
  Sum2/1 -> Gain1/1
  "Value heat exchange outdoor -> rooms"/1(Q_outdoor_to_rooms) -> Sum2/2
  T_rooms/1 -> "Value heat exchange outdoor -> rooms"/1(T_rooms), Value heat exchange within building/1("T_rooms ")
  T_outdoor/1 -> "Value heat exchange outdoor -> rooms"/2(outdoor)
  Gain7/1 -> "Delta_wall_rooms "/1
  Value heat exchange within building/1(Q_in_building_to_rooms) -> Sum2/1

== system model_socrates/Subsystem/Energy consumption air conditionners (per private rooms) ==
  note: Energy used by air conditionners in the private rooms
  air_conditionner_on_off : Inport
  Data Type Conversion : DataTypeConversion
  Gain : Gain  Gain=nb_second_in_timeunit
  Gain3 : Gain  Gain=Energy_used_by_air_conditioner_for_1_timeunit_in_Watts_vector
  Sum : Sum  Inputs=|++
  Unit Delay : UnitDelay  SampleTime=-1  HasFrameUpgradeWarning=on
  energy_used_by_air_cons_per_private_room_(vector) : Outport
  wires:
  Gain3/1 -> Gain/1
  Sum/1 -> Unit Delay/1
  air_conditionner_on_off/1 -> Data Type Conversion/1
  Unit Delay/1 -> Sum/2, Gain3/1
  Data Type Conversion/1 -> Sum/1
  Gain/1 -> energy_used_by_air_cons_per_private_room_(vector)/1

== system model_socrates/Subsystem/Energy consumption air mixer ==
  note: Ventilation energy consumption
  Constant : Constant
  Gain : Gain  Gain=nb_second_in_timeunit
  Gain3 : Gain  Gain=Energy_used_by_air_mixer_for_1_timeunit_in_Watts
  Sum : Sum  Inputs=|++
  Unit Delay : UnitDelay  SampleTime=-1  HasFrameUpgradeWarning=on
  Energy_used_by_air_mixer : Outport
  wires:
  Gain3/1 -> Gain/1
  Sum/1 -> Unit Delay/1
  Unit Delay/1 -> Gain3/1, Sum/2
  Constant/1 -> Sum/1
  Gain/1 -> Energy_used_by_air_mixer/1

== system model_socrates/Subsystem/Energy consumption boiler ==
  note: Energy consumption of the boiler
  Boiler_on_off : Inport
  Data Type Conversion : DataTypeConversion
  Gain : Gain  Gain=nb_second_in_timeunit
  Gain3 : Gain  Gain=Energy_used_by_boiler_for_1_timeunit_in_Watts
  Sum : Sum  Inputs=|++
  Unit Delay : UnitDelay  SampleTime=-1  HasFrameUpgradeWarning=on
  Energy_used_by_boiler : Outport
  wires:
  Data Type Conversion/1 -> Sum/1
  Sum/1 -> Unit Delay/1
  Unit Delay/1 -> Gain3/1, Sum/2
  Gain3/1 -> Gain/1
  Boiler_on_off/1 -> Data Type Conversion/1
  Gain/1 -> Energy_used_by_boiler/1

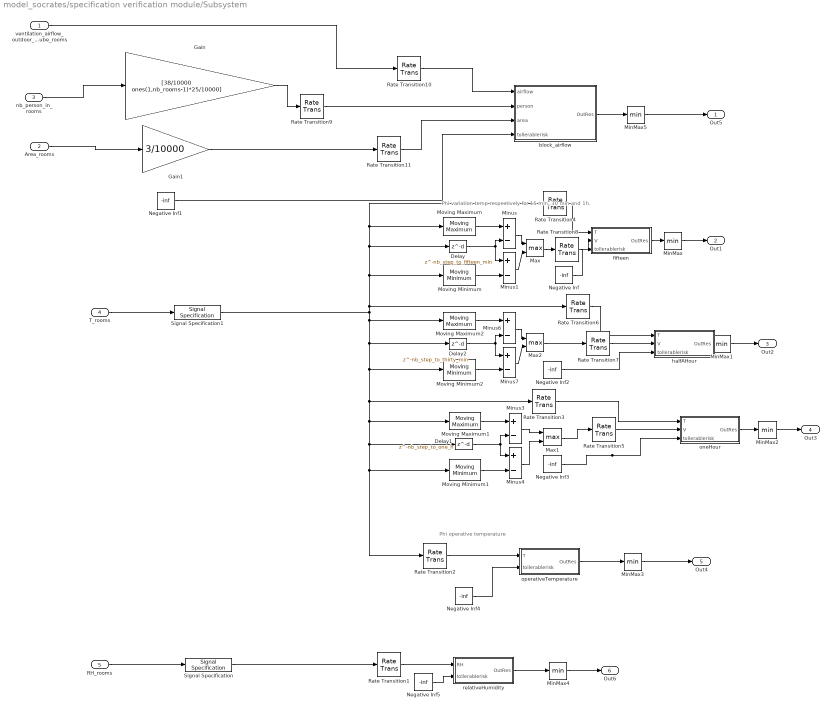
== system model_socrates/specification verification module/Subsystem ==
  note: Phi variation temp respectively for 15 min, 30 min and 1h.
  note: Phi operative temperature
  ventilation_airflow_outdoor_air_mcube_rooms : Inport  PortDimensions=nb_rooms
  Area_rooms : Inport  Port=2  PortDimensions=nb_rooms
  nb_person_in_rooms : Inport  Port=3  OutDataTypeStr=double  PortDimensions=nb_rooms
  T_rooms : Inport  Port=4  PortDimensions=nb_rooms
  RH_rooms : Inport  Port=5  PortDimensions=nb_rooms
  Delay : Delay  DelayLength=nb_step_to_fifteen_min  InitialCondition=27
  Delay1 : Delay  DelayLength=nb_step_to_one_h  InitialCondition=27
  Delay2 : Delay  DelayLength=nb_step_to_thirty_min  InitialCondition=27
  Gain : Gain  Gain=[38/10000 ones(1,nb_rooms-1)*25/10000]
  Gain1 : Gain  Gain=3/10000
  Max : MinMax  Function=max  Inputs=2  ZeroCross=off
  Max1 : MinMax  Function=max  Inputs=2  ZeroCross=off
  Max2 : MinMax  Function=max  Inputs=2  ZeroCross=off
  MinMax{,1..5} (6 alike) : MinMax
  Minus{,1,3..4,6..7} (6 alike) : Sum  Inputs=+-
  Moving Maximum : dspstat3/Moving Maximum  SpecifyWindowLength=on  WindowLength=nb_step_to_fifteen_min  SimulateUsing=Code generation
      settings: SourceProductName=DSP System Toolbox  SourceProductBaseCode=DS
  Moving Maximum1 : dspstat3/Moving Maximum  SpecifyWindowLength=on  WindowLength=nb_step_to_one_h  SimulateUsing=Code generation
      settings: SourceProductName=DSP System Toolbox  SourceProductBaseCode=DS
  Moving Maximum2 : dspstat3/Moving Maximum  SpecifyWindowLength=on  WindowLength=nb_step_to_thirty_min  SimulateUsing=Code generation
      settings: SourceProductName=DSP System Toolbox  SourceProductBaseCode=DS
  Moving Minimum : dspstat3/Moving Minimum  SpecifyWindowLength=on  WindowLength=nb_step_to_fifteen_min  SimulateUsing=Code generation
      settings: SourceProductName=DSP System Toolbox  SourceProductBaseCode=DS
  Moving Minimum1 : dspstat3/Moving Minimum  SpecifyWindowLength=on  WindowLength=nb_step_to_one_h  SimulateUsing=Code generation
      settings: SourceProductName=DSP System Toolbox  SourceProductBaseCode=DS
  Moving Minimum2 : dspstat3/Moving Minimum  SpecifyWindowLength=on  WindowLength=nb_step_to_thirty_min  SimulateUsing=Code generation
      settings: SourceProductName=DSP System Toolbox  SourceProductBaseCode=DS
  Negative Inf{,1..5} (6 alike) : Constant  Value=-inf  OutDataTypeStr=Inherit: Inherit via back propagation
  Rate Transition{1..11} (11 alike) : RateTransition  OutPortSampleTime=rate
  Signal Specification : SignalSpecification  OutMin=-0.25  OutMax=1.25  Dimensions=nb_rooms
  Signal Specification1 : SignalSpecification  OutMin=-100  OutMax=100  Dimensions=nb_rooms
  block_airflow : Subsystem
  fifteen : Subsystem
  halfAHour : Subsystem
  oneHour : Subsystem
  operativeTemperature : Subsystem
  relativeHumidity : Subsystem
  Out5 : Outport
  Out1 : Outport  Port=2
  Out2 : Outport  Port=3
  Out3 : Outport  Port=4
  Out4 : Outport  Port=5
  Out6 : Outport  Port=6
  wires:
  Minus4/1 -> Max1/2
  Moving Minimum1/1 -> Minus4/2
  Negative Inf2/1 -> halfAHour/3(tollerablerisk)
  Rate Transition6/1 -> halfAHour/1(T)
  Delay2/1 -> Minus6/2, Minus7/1
  MinMax5/1 -> Out5/1
  ventilation_airflow_outdoor_air_mcube_rooms/1 -> Rate Transition10/1
  MinMax4/1 -> Out6/1
  Rate Transition7/1 -> halfAHour/2(V)
  Negative Inf5/1 -> relativeHumidity/2(tollerablerisk)
  Minus3/1 -> Max1/1
  Moving Maximum2/1 -> Minus6/1
  MinMax3/1 -> Out4/1
  Rate Transition10/1 -> block_airflow/1(airflow)
  MinMax2/1 -> Out3/1
  MinMax1/1 -> Out2/1
  Moving Maximum/1 -> Minus/1
  Rate Transition8/1 -> fifteen/2(V)
  Delay/1 -> Minus1/1, Minus/2
  Rate Transition5/1 -> oneHour/2(V)
  nb_person_in_rooms/1 -> Gain/1
  Max/1 -> Rate Transition8/1
  Area_rooms/1 -> Gain1/1
  Negative Inf1/1 -> block_airflow/4(tollerablerisk)
  Minus6/1 -> Max2/1
  Minus/1 -> Max/1
  oneHour/1(OutRes) -> MinMax2/1
  Gain1/1 -> Rate Transition11/1
  Max2/1 -> Rate Transition7/1
  RH_rooms/1 -> Signal Specification/1
  T_rooms/1 -> Signal Specification1/1
  Negative Inf/1 -> fifteen/3(tollerablerisk)
  Rate Transition3/1 -> oneHour/1(T)
  operativeTemperature/1(OutRes) -> MinMax3/1
  block_airflow/1(OutRes) -> MinMax5/1
  Rate Transition11/1 -> block_airflow/3(area)
  relativeHumidity/1(OutRes) -> MinMax4/1
  Signal Specification/1 -> Rate Transition1/1
  halfAHour/1(OutRes) -> MinMax1/1
  Minus7/1 -> Max2/2
  MinMax/1 -> Out1/1
  fifteen/1(OutRes) -> MinMax/1
  Negative Inf4/1 -> operativeTemperature/2(tollerablerisk)
  Moving Minimum2/1 -> Minus7/2
  Moving Minimum/1 -> Minus1/2
  Signal Specification1/1 -> Rate Transition2/1, Moving Minimum1/1, Delay1/1, Moving Maximum1/1, Rate Transition3/1, Moving Minimum2/1, Delay2/1, Moving Maximum2/1, Rate Transition6/1, Rate Transition4/1, Moving Maximum/1, Delay/1, Moving Minimum/1
  Moving Maximum1/1 -> Minus3/1
  Gain/1 -> Rate Transition9/1
  Rate Transition1/1 -> relativeHumidity/1(RH)
  Max1/1 -> Rate Transition5/1
  Negative Inf3/1 -> oneHour/3(tollerablerisk)
  Rate Transition4/1 -> fifteen/1(T)
  Rate Transition2/1 -> operativeTemperature/1(T)
  Rate Transition9/1 -> block_airflow/2(person)
  Delay1/1 -> Minus3/2, Minus4/1
  Minus1/1 -> Max/2
